simulink model "inverted_pendulum_sim_fuz_dk"  (R2021a)
settings: Solver=VariableStepAuto  StartTime=0.0  StopTime=10  RelTol=1e-3
values from neighbouring files (symbols this model uses):
  g = 9.8    [inverted_pendulum_fuz.m]
  L = 0.12    [inverted_pendulum_fuz.m]
  m = 0.017    [inverted_pendulum_fuz.m]
  M = 0.07    [inverted_pendulum_fuz.m]
  Mm = 20*0.001    (= 0.02)    [inverted_pendulum_fuz.m]
  R = 0.065    [inverted_pendulum_fuz.m]
  Rm = 26.3/2*0.01    (= 0.1315)    [inverted_pendulum_fuz.m]
  theta1_ini = pi*(20)/180    (= 0.349065850399)    [inverted_pendulum_fuz.m]
libraries: fuzblock x1
settings Model: Creator=18214  LastModifiedBy=18214

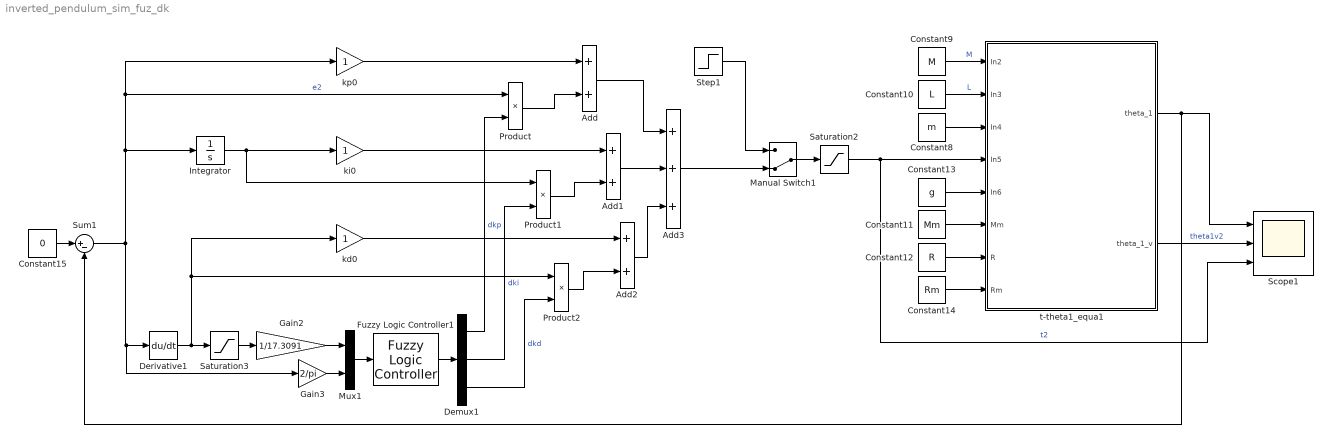
== system inverted_pendulum_sim_fuz_dk ==
  Add : Sum
  Add1 : Sum
  Add2 : Sum
  Add3 : Sum  Inputs=+++
  Constant10 : Constant  Value=L
  Constant11 : Constant  Value=Mm
  Constant12 : Constant  Value=R
  Constant13 : Constant  Value=g
  Constant14 : Constant  Value=Rm
  Constant15 : Constant  Value=0
  Constant8 : Constant  Value=m
  Constant9 : Constant  Value=M
  Demux1 : Demux  Outputs=3
  Derivative1 : Derivative
  Fuzzy Logic Controller1 : fuzblock/Fuzzy Logic  Controller  FIS='fuzzyctr.fis'  OutputSampleNumber=101  DataType=double  FuzzifiedInputs=off  RuleFiringStrengths=off  RuleOutputs=off  AggregatedOutputs=off  SimulateUsing=Interpreted execution  OutOfRangeInputValueMessage=warning  NoRuleFiredMessage=warning  EmptyOutputFuzzySetMessage=warning
  Gain2 : Gain  Gain=1/17.3091
  Gain3 : Gain  Gain=2/pi
  Integrator : Integrator
  Manual Switch1 : ManualSwitch  CurrentSetting=0
  Mux1 : Mux  Inputs=2
  Product : Product
  Product1 : Product
  Product2 : Product
  Saturation2 : Saturate  UpperLimit=inf  LowerLimit=-inf
  Saturation3 : Saturate  UpperLimit=17.3091  LowerLimit=-17.3091
  Scope1 : Scope  NumInputPorts=3
  Step1 : Step  After=0  SampleTime=0
  Sum1 : Sum  Inputs=|+-
  kd0 : Gain
  ki0 : Gain
  kp0 : Gain
  t-theta1_equa1 : Subsystem
  wires:
  Product1/1 -> Add1/2
  kd0/1 -> Add2/1
  ki0/1 -> Add1/1
  Product/1 -> Add/2
  kp0/1 -> Add/1
  Constant9/1 -> t-theta1_equa1/1(In2)  "M"
  Add1/1 -> Add3/2
  Sum1/1 -> Integrator/1, Product/1, kp0/1, Gain3/1, Derivative1/1  "e2"
  Constant12/1 -> t-theta1_equa1/7(R)
  Manual Switch1/1 -> Saturation2/1
  Saturation2/1 -> t-theta1_equa1/4(In5), Scope1/3  "t2"
  Constant15/1 -> Sum1/1
  Mux1/1 -> Fuzzy Logic Controller1/1
  t-theta1_equa1/2(theta_1_v) -> Scope1/2  "theta1v2"
  Add3/1 -> Manual Switch1/2
  Saturation3/1 -> Gain2/1
  Constant13/1 -> t-theta1_equa1/5(In6)
  Constant11/1 -> t-theta1_equa1/6(Mm)
  Step1/1 -> Manual Switch1/1
  Gain3/1 -> Mux1/2
  Gain2/1 -> Mux1/1
  Fuzzy Logic Controller1/1 -> Demux1/1
  Constant8/1 -> t-theta1_equa1/3(In4)
  Constant14/1 -> t-theta1_equa1/8(Rm)
  Constant10/1 -> t-theta1_equa1/2(In3)  "L"
  Integrator/1 -> Product1/1, ki0/1
  Add/1 -> Add3/1
  Product2/1 -> Add2/2
  Demux1/2 -> Product1/2  "dki"
  t-theta1_equa1/1(theta_1) -> Scope1/1, Sum1/2
  Demux1/1 -> Product/2  "dkp"
  Add2/1 -> Add3/3
  Demux1/3 -> Product2/2  "dkd"
  Derivative1/1 -> Product2/1, kd0/1, Saturation3/1

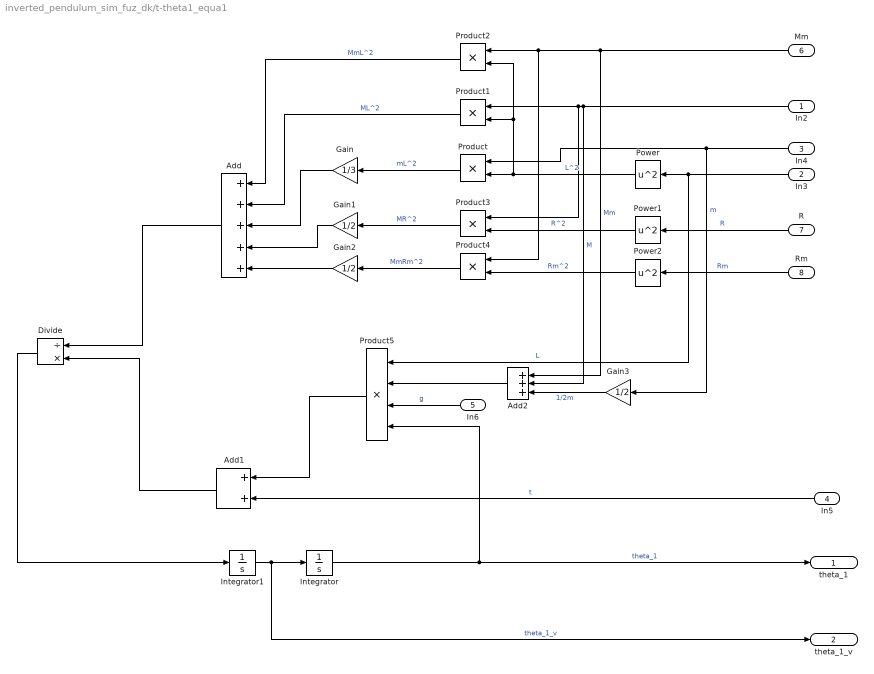
== system inverted_pendulum_sim_fuz_dk/t-theta1_equa1 ==
  In2 : Inport
  In3 : Inport  Port=2
  In4 : Inport  Port=3
  In5 : Inport  Port=4
  In6 : Inport  Port=5
  Mm : Inport  Port=6
  R : Inport  Port=7
  Rm : Inport  Port=8
  Add : Sum  Inputs=+++++
  Add1 : Sum
  Add2 : Sum  Inputs=+++
  Divide : Product  Inputs=/*
  Gain : Gain  Gain=1/3
  Gain1 : Gain  Gain=1/2
  Gain2 : Gain  Gain=1/2
  Gain3 : Gain  Gain=1/2
  Integrator : Integrator  InitialCondition=theta1_ini  LowerSaturationLimit=-pi
  Integrator1 : Integrator
  Power : Math  Operator=square  SaturateOnIntegerOverflow=on
  Power1 : Math  Operator=square  SaturateOnIntegerOverflow=on
  Power2 : Math  Operator=square  SaturateOnIntegerOverflow=on
  Product{,1..4} (5 alike) : Product
  Product5 : Product  Inputs=4
  theta_1 : Outport
  theta_1_v : Outport  Port=2
  wires:
  Integrator/1 -> Product5/4, theta_1/1  "theta_1"
  Integrator1/1 -> theta_1_v/1, Integrator/1  "theta_1_v"
  Mm/1 -> Product4/1, Product2/1, Add2/1  "Mm"
  R/1 -> Power1/1  "R"
  Rm/1 -> Power2/1  "Rm"
  In3/1 -> Product5/1, Power/1  "L"
  Power/1 -> Product2/2, Product1/2, Product/2  "L^2"
  In4/1 -> Product/1, Gain3/1  "m"
  Product/1 -> Gain/1  "mL^2"
  In2/1 -> Product1/1, Product3/1, Add2/2  "M"
  Product1/1 -> Add/2  "ML^2"
  Product2/1 -> Add/1  "MmL^2"
  Power1/1 -> Product3/2  "R^2"
  Power2/1 -> Product4/2  "Rm^2"
  Product3/1 -> Gain1/1  "MR^2"
  Product4/1 -> Gain2/1  "MmRm^2"
  Gain2/1 -> Add/5
  Gain1/1 -> Add/4
  Gain/1 -> Add/3
  Add/1 -> Divide/1
  Add1/1 -> Divide/2
  In5/1 -> Add1/2  "t"
  Gain3/1 -> Add2/3  "1/2m"
  Add2/1 -> Product5/2
  In6/1 -> Product5/3  "g"
  Divide/1 -> Integrator1/1
  Product5/1 -> Add1/1
